simulink model "TST_LogicOperations"  (Simulink 7.4)
settings: Solver=FixedStepDiscrete  StartTime=0.0  StopTime=10.0  FixedStep=0.02  RelTol=1e-3
settings Model: Creator=kharthforeign  LastModifiedBy=kharthforeign  BufferReuse=off
settings DataIOCC: SaveOutput=off  SignalLogging=off  SaveTime=off
settings OptimizationCC: BlockReduction=off  ConditionallyExecuteInputs=off  OptimizeBlockIOStorage=off  BufferReuse=off  ExpressionFolding=off  LocalBlockOutputs=off  InitFltsAndDblsToZero=on

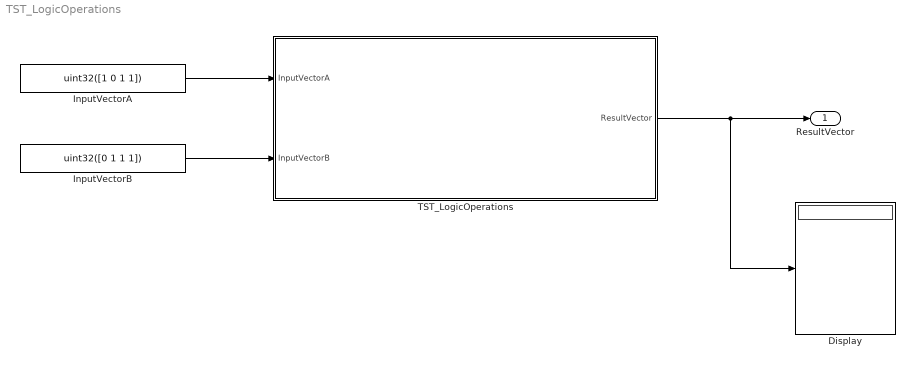
== system TST_LogicOperations ==
  Display : Display
  InputVectorA : Constant  Value=uint32([1 0 1 1])  OutDataType=fixdt(1, 16)  OutScaling=2^0
  InputVectorB : Constant  Value=uint32([0 1 1 1])  OutDataType=fixdt(1, 16)  OutScaling=2^0
  TST_LogicOperations : Subsystem  TreatAsAtomicUnit=on
  ResultVector : Outport  OutDataType=fixdt(1, 16)  OutScaling=2^0
  wires:
  TST_LogicOperations/1(ResultVector) -> ResultVector/1, Display/1
  InputVectorA/1 -> TST_LogicOperations/1(InputVectorA)
  InputVectorB/1 -> TST_LogicOperations/2(InputVectorB)

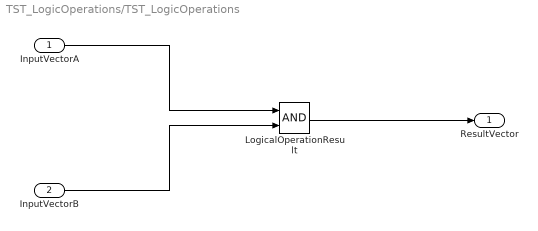
== system TST_LogicOperations/TST_LogicOperations ==
  InputVectorA : Inport  OutDataType=fixdt(1, 16)  OutScaling=2^0
  InputVectorB : Inport  Port=2  OutDataType=fixdt(1, 16)  OutScaling=2^0
  LogicalOperationResult : Logic  AllPortsSameDT=off  OutDataTypeMode=boolean  LogicDataType=fixdt(0, 8)  OutDataTypeStr=boolean
  ResultVector : Outport  OutDataType=fixdt(1, 16)  OutScaling=2^0
  wires:
  InputVectorA/1 -> LogicalOperationResult/1
  InputVectorB/1 -> LogicalOperationResult/2
  LogicalOperationResult/1 -> ResultVector/1
